simulink model "CrystallizationModel"  (R2024a)
settings: Solver=VariableStepAuto  StartTime=0.0  StopTime=10.0  RelTol=1e-3
libraries: simulink x1
settings Model: Creator=User  LastModifiedBy=User

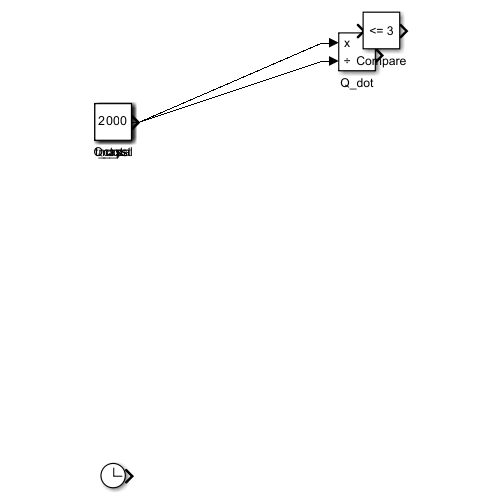
[thumbnail: Simulink's stored preview of the top-level diagram]
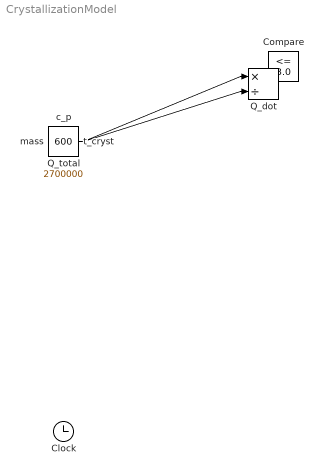
== system CrystallizationModel ==
  Clock : Clock
  Compare : simulink/Logic and Bit Operations/Compare To Constant  relop=<=  const=3.0  OutDataTypeStr=boolean
  Q_dot : Product  Inputs=*/
  Q_total : Constant  Value=2700000
  c_p : Constant  Value=2000
  mass : Constant  Value=9.4
  t_cryst : Constant  Value=600
  wires:
  Q_total/1 -> Q_dot/1
  t_cryst/1 -> Q_dot/2
